simulink model "rectifiers"  (R2016a)
settings: Solver=ode4  StartTime=0.0  StopTime=2  FixedStep=1e-5  RelTol=1e-3
undefined symbols (not defined in the file): D1, lagging, pulse
libraries: powerlib x34, powerlib_meascontrol x20
settings Model: Creator=ugurm  LastModifiedBy=mesutto
settings DataIOCC: LimitDataPoints=on  SaveFormat=Array
settings DebuggingCC: UnderspecifiedInitializationDetection=Classic  MergeDetectMultiDrivingBlocksExec=none  SolverPrmCheckMsg=warning  StateNameClashWarn=warning
settings HardwareCC: ProdBitPerPointer=32  ProdLargestAtomicFloat=None  ProdIntDivRoundTo=Undefined  ProdEndianess=Unspecified  ProdWordSize=32  ProdHWDeviceType=32-bit Generic
settings ModelReferenceCC: PropagateSignalLabelsOutOfModel=off
settings ConfigComp: CovModelRefEnable=Off

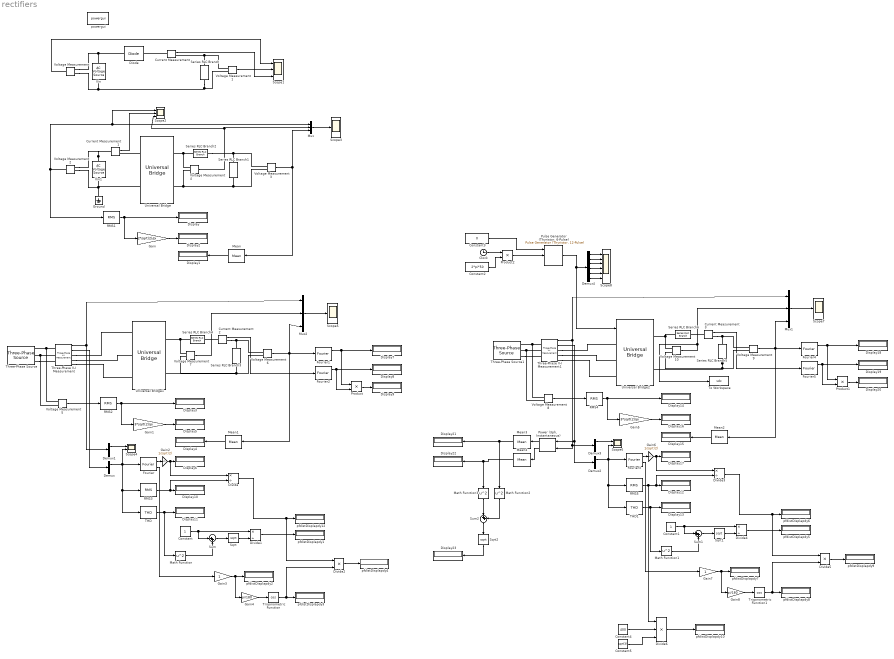
== system rectifiers ==
  Clock : Clock
  Constant : Constant
  Constant1 : Constant
  Constant2 : Constant  Value=2*pi*50
  Constant3 : Constant  Value=0
  Constant4 : Constant  Value=400
  Constant5 : Constant  Value=sqrt(3)
  Current Measurement{,1..3} (4 alike) : powerlib/Measurements/Current Measurement  PhasorSimulation=off  OutputType=Complex  PSBequivalent=0
  Demux{,1..3} (4 alike) : Demux  Outputs=3
  Demux4 : Demux  Outputs=6
  Diode : powerlib/Power Electronics/Diode  Ron=0.001  Lon=0  Vf=0.8  IC=0  UseSnubber=off  Rs=1e9  Cs=250e-9  Measurements=off
  Display{,1..23} (24 alike) : Display
  Divide{,1,3..4} (4 alike) : Product  Inputs=*/
  Divide2 : Product  Inputs=**
  Divide5 : Product  Inputs=**
  Divide6 : Product  Inputs=***
  Fourier : powerlib_meascontrol/Measurements/Fourier  Freq=50  n=1  InInit=[0, 0]  Ts=0
  Fourier{1..2,4..5} (4 alike) : powerlib_meascontrol/Measurements/Fourier  Freq=50  n=0  InInit=[0, 0]  Ts=0
  Fourier3 : powerlib_meascontrol/Measurements/Fourier  Freq=50  n=1  InInit=[0, 0]  Ts=0
  Gain : Gain  Gain=2*sqrt(2)/pi
  Gain1 : Gain  Gain=3*sqrt(2)/pi
  Gain2 : Gain  Gain=1/sqrt(2)
  Gain3 : Gain
  Gain4 : Gain  Gain=pi/180
  Gain5 : Gain  Gain=3*sqrt(2)/pi
  Gain6 : Gain  Gain=1/sqrt(2)
  Gain7 : Gain
  Gain8 : Gain  Gain=pi/180
  Ground : powerlib/Elements/Ground  LConnTagsString=a
  Math Function{,1..3} (4 alike) : Math  Operator=square  SaturateOnIntegerOverflow=on
  Mean{,1..4} (5 alike) : powerlib_meascontrol/Measurements/Mean  Freq=50  Vinit=0  Ts=0
  Mux : Mux  Inputs=3
  Mux1 : Mux  Inputs=3
  Mux2 : Mux  Inputs=3
  "Power (3ph, Instantaneous)" : powerlib_meascontrol/Measurements/Power (3ph, Instantaneous)
  Product : Product
  Product1 : Product
  Product2 : Product
  "Pulse Generator (Thyristor, 6-Pulse)" : powerlib_meascontrol/Pulse & Signal Generators/Pulse Generator (Thyristor, 12-Pulse)  GenType=6-pulse  Delta=D1 (lagging)  pwidth=60  Double_Pulse=off  Ts=0
  RMS{1..5} (5 alike) : powerlib_meascontrol/Measurements/RMS  TrueRMS=on  Freq=50  RMSInit=0  Ts=0
  Scope1 : Scope  NumInputPorts=3
  Scope2 : Scope  NumInputPorts=3
  Scope3 : Scope
  Scope4 : Scope  NumInputPorts=2
  Scope5 : Scope
  Scope6 : Scope  NumInputPorts=2
  Scope7 : Scope
  Scope8 : Scope  NumInputPorts=6
  Series RLC Branch : powerlib/Elements/Series RLC Branch  LConnTagsString=__new0  RConnTagsString=__new0  BranchType=RL  Resistance=2  Inductance=1/(2*pi*50)  SetiL0=off  InitialCurrent=0  Capacitance=1e-6  Setx0=off  InitialVoltage=0  Measurements=None
  Series RLC Branch1 : powerlib/Elements/Series RLC Branch  LConnTagsString=__new0  RConnTagsString=__new0  BranchType=R  Resistance=2  Inductance=1/(2*pi*50)  SetiL0=off  InitialCurrent=0  Capacitance=1e-6  Setx0=off  InitialVoltage=0  Measurements=None
  Series RLC Branch2 : powerlib/Elements/Series RLC Branch  LConnTagsString=__new0  RConnTagsString=__new0  BranchType=L  Resistance=2  Inductance=100/(2*pi*50)  SetiL0=off  InitialCurrent=0  Capacitance=1e-6  Setx0=off  InitialVoltage=0  Measurements=None
  Series RLC Branch3 : powerlib/Elements/Series RLC Branch  LConnTagsString=__new0  RConnTagsString=__new0  BranchType=R  Resistance=54  Inductance=1/(2*pi*50)  SetiL0=off  InitialCurrent=0  Capacitance=1e-6  Setx0=off  InitialVoltage=0  Measurements=None
  Series RLC Branch4 : powerlib/Elements/Series RLC Branch  LConnTagsString=__new0  RConnTagsString=__new0  BranchType=L  Resistance=2  Inductance=100/(2*pi*50)  SetiL0=off  InitialCurrent=0  Capacitance=1e-6  Setx0=off  InitialVoltage=0  Measurements=None
  Series RLC Branch5 : powerlib/Elements/Series RLC Branch  LConnTagsString=__new0  RConnTagsString=__new0  BranchType=R  Resistance=5  Inductance=1/(2*pi*50)  SetiL0=off  InitialCurrent=0  Capacitance=1e-6  Setx0=off  InitialVoltage=0  Measurements=None
  Series RLC Branch6 : powerlib/Elements/Series RLC Branch  LConnTagsString=__new0  RConnTagsString=__new0  BranchType=L  Resistance=2  Inductance=100/(2*pi*50)  SetiL0=off  InitialCurrent=0  Capacitance=1e-6  Setx0=off  InitialVoltage=0  Measurements=None
  Sqrt : Sqrt  SaturateOnIntegerOverflow=on
  Sqrt1 : Sqrt  SaturateOnIntegerOverflow=on
  Sqrt2 : Sqrt  SaturateOnIntegerOverflow=on
  Sum : Sum  Inputs=|++
  Sum1 : Sum  Inputs=|++
  Sum2 : Sum  Inputs=|++
  THD : powerlib_meascontrol/Measurements/THD  Freq=50  Ts=0
  THD1 : powerlib_meascontrol/Measurements/THD  Freq=50  Ts=0
  Three-Phase V-I Measurement : powerlib/Measurements/Three-Phase V-I Measurement  VoltageMeasurement=phase-to-ground  SetLabelV=off  LabelV=Vabc  Vpu=off  VpuLL=off  CurrentMeasurement=yes  SetLabelI=off  LabelI=Iabc  Ipu=off  Pbase=100e6  Vbase=500e3  OutputType=Complex  PhasorSimulation=off  PSBequivalent=0
  Three-Phase V-I Measurement1 : powerlib/Measurements/Three-Phase V-I Measurement  VoltageMeasurement=phase-to-ground  SetLabelV=off  LabelV=Vabc  Vpu=off  VpuLL=off  CurrentMeasurement=yes  SetLabelI=off  LabelI=Iabc  Ipu=off  Pbase=100e6  Vbase=500e3  OutputType=Complex  PhasorSimulation=off  PSBequivalent=0
  Three-Phase Source : powerlib/Electrical Sources/Three-Phase Source  InternalConnection=Yg  VoltagePhases=off  Voltage=400  PhaseAngle=0  Voltage_phases=[25e3 25e3 25e3]/sqrt(3)  PhaseAngles_phases=[0 -120 +120]  Frequency=50  NonIdealSource=off  SpecifyImpedance=off  Resistance=0.8929  Inductance=16.58e-3  ShortCircuitLevel=100e6  BaseVoltage=25e3  XRratio=7  BusType=swing  Pref=10e3  Qref=0  Prefabc=[10e3, 10e3, 10e3]  Qrefabc=[0, 0, 0]  Qmin=-inf  Qmax=inf
  Three-Phase Source1 : powerlib/Electrical Sources/Three-Phase Source  InternalConnection=Yg  VoltagePhases=off  Voltage=400  PhaseAngle=0  Voltage_phases=[25e3 25e3 25e3]/sqrt(3)  PhaseAngles_phases=[0 -120 +120]  Frequency=50  NonIdealSource=off  SpecifyImpedance=off  Resistance=0.8929  Inductance=16.58e-3  ShortCircuitLevel=100e6  BaseVoltage=25e3  XRratio=7  BusType=swing  Pref=10e3  Qref=0  Prefabc=[10e3, 10e3, 10e3]  Qrefabc=[0, 0, 0]  Qmin=-inf  Qmax=inf
  To Workspace : ToWorkspace  VariableName=vdc  SaveFormat=Structure With Time  SampleTime=-1
  Trigonometric Function : Trigonometry  Operator=cos
  Trigonometric Function1 : Trigonometry  Operator=cos
  Universal Bridge : powerlib/Power Electronics/Universal Bridge  Arms=2  SnubberResistance=1e5  SnubberCapacitance=inf  Device=Diodes  Ron=1e-3  Lon=0  ForwardVoltages="[  0  0  ]"  ForwardVoltage=0  GTOparameters=[ 10e-6 , 20e-6 ]  IGBTparameters=[ 1e-6 , 2e-6 ]  Measurements=None  Measurements_2=None  converterType=Rectifier
  Universal Bridge1 : powerlib/Power Electronics/Universal Bridge  Arms=3  SnubberResistance=1e5  SnubberCapacitance=inf  Device=Diodes  Ron=1e-3  Lon=0  ForwardVoltages="[  0  0  ]"  ForwardVoltage=0  GTOparameters=[ 10e-6 , 20e-6 ]  IGBTparameters=[ 1e-6 , 2e-6 ]  Measurements=None  Measurements_2=None  converterType=Rectifier
  Universal Bridge2 : powerlib/Power Electronics/Universal Bridge  Arms=3  SnubberResistance=1e5  SnubberCapacitance=inf  Device=Thyristors  Ron=1e-3  Lon=0  ForwardVoltages="[  0  0  ]"  ForwardVoltage=0  GTOparameters=[ 10e-6 , 20e-6 ]  IGBTparameters=[ 1e-6 , 2e-6 ]  Measurements=None  Measurements_2=None  converterType=Rectifier
  Vin : powerlib/Electrical Sources/AC Voltage Source  Amplitude=230*sqrt(2)  Phase=0  Frequency=50  SampleTime=0  Measurements=None  BusType=swing  Pref=10e3  Qref=0  Qmin=-inf  Qmax=+inf
  Vin1 : powerlib/Electrical Sources/AC Voltage Source  Amplitude=230*sqrt(2)  Phase=0  Frequency=50  SampleTime=0  Measurements=None  BusType=swing  Pref=10e3  Qref=0  Qmin=-inf  Qmax=+inf
  Voltage Measurement{,1..10} (11 alike) : powerlib/Measurements/Voltage Measurement  PhasorSimulation=off  OutputType=Complex  PSBequivalent=0
  pfdistDisplapdy{1..10,12} (11 alike) : Display
  powergui : powerlib/powergui  Priority=1  SimulationMode=Discrete  SolverType=Tustin/Backward Euler (TBE)  SampleTime=1e-5  frequency=60  SPID=off  DisableSnubberDevices=off  DisableRonSwitches=off  DisableVfSwitches=off  SwTol=0  DisplayEquations=off  Interpol=off  ExternalGateDelay=off  methode=off  Ts=10  FunctionMessages=off  echomessages=off  HookPort=off  EnableUseOfTLC=off  x0status=blocks  frequencyindice=50  Pbase=100e6  ErrMax=1e-4  Iterations=50  UnitsV=kV  UnitsW=MW  buscounter=0  RestoreLinks=warning  ResistiveCurrentMeasurement=off  Frange=[0:2:500]  Ylog=off  Xlog=on  ShowGrid=off  save=off  variable=ZData  structure=vdc  ZoomFFT=off  StartTime=0.2  cycles=20  DisplayStyle=5  fundamental=50  FreqAxis=off  MaxFrequency=2000  frequencyindicesteady=1  RmsSteady=1  display=off
  wires:
  Voltage Measurement/1 -> Scope1/1
  Voltage Measurement1/1 -> Scope1/2
  Current Measurement/1 -> Scope1/3
  Voltage Measurement2/1 -> Scope2/1, Mux/1, RMS1/1
  Voltage Measurement4/1 -> Scope2/3, Mux/2
  Voltage Measurement3/1 -> Mux/3, Mean/1
  Mux/1 -> Scope3/1
  RMS1/1 -> Gain/1, Display/1
  Current Measurement1/1 -> Scope2/2
  Mean/1 -> Display1/1
  Gain/1 -> Display2/1
  Voltage Measurement6/1 -> Mux2/3, Mean1/1, Fourier1/1
  RMS2/1 -> Gain1/1, Display3/1
  Mean1/1 -> Display4/1
  Gain1/1 -> Display5/1
  Three-Phase V-I Measurement/1 -> Demux1/1, Mux2/1
  Voltage Measurement7/1 -> Mux2/2
  Mux2/1 -> Scope5/1
  Voltage Measurement5/1 -> RMS2/1
  Three-Phase V-I Measurement/2 -> Demux/1
  Demux/1 -> THD/1, RMS3/1, Scope4/2, Fourier/1
  Fourier/1 -> Gain2/1
  Current Measurement2/1 -> Fourier2/1
  Fourier1/1 -> Product/1, Display7/1
  Fourier2/1 -> Product/2, Display8/1
  Product/1 -> Display9/1
  Demux1/1 -> Scope4/1
  RMS3/1 -> Divide/2, Display10/1
  Gain2/1 -> Divide/1, Display6/1
  THD/1 -> Math Function/1, Display11/1
  Divide/1 -> Divide2/1, pfdistDisplapdy12/1
  Constant/1 -> Sum/1, Divide1/1
  Sqrt/1 -> Divide1/2
  Math Function/1 -> Sum/2
  Sum/1 -> Sqrt/1
  Divide1/1 -> pfdistDisplapdy1/1
  Fourier/2 -> Gain3/1
  Gain3/1 -> Gain4/1, pfdistDisplapdy2/1
  Trigonometric Function/1 -> Divide2/2, pfdistDisplapdy3/1
  Divide2/1 -> pfdistDisplapdy4/1
  Gain4/1 -> Trigonometric Function/1
  Voltage Measurement9/1 -> Mux1/3, Mean2/1, Fourier4/1
  RMS4/1 -> Gain5/1, Display14/1
  Mean2/1 -> Display15/1
  Gain5/1 -> Display16/1
  Three-Phase V-I Measurement1/1 -> "Power (3ph, Instantaneous)"/1, Demux3/1, Mux1/1
  Voltage Measurement10/1 -> To Workspace/1, Mux1/2
  Mux1/1 -> Scope7/1
  Voltage Measurement8/1 -> RMS4/1
  Three-Phase V-I Measurement1/2 -> Demux2/1, "Power (3ph, Instantaneous)"/2
  Demux2/1 -> THD1/1, RMS5/1, Scope6/2, Fourier3/1
  Fourier3/1 -> Gain6/1
  Current Measurement3/1 -> Fourier5/1
  Fourier4/1 -> Product1/1, Display18/1
  Fourier5/1 -> Product1/2, Display19/1
  Product1/1 -> Display20/1
  Demux3/1 -> Scope6/1
  RMS5/1 -> Divide6/1, Divide3/2, Display12/1
  Gain6/1 -> Divide3/1, Display17/1
  THD1/1 -> Math Function1/1, Display13/1
  Divide3/1 -> Divide5/1, pfdistDisplapdy6/1
  Constant1/1 -> Sum1/1, Divide4/1
  Sqrt1/1 -> Divide4/2
  Math Function1/1 -> Sum1/2
  Sum1/1 -> Sqrt1/1
  Divide4/1 -> pfdistDisplapdy5/1
  Fourier3/2 -> Gain7/1
  Gain7/1 -> Gain8/1, pfdistDisplapdy7/1
  Trigonometric Function1/1 -> Divide5/2, pfdistDisplapdy8/1
  Divide5/1 -> pfdistDisplapdy9/1
  Gain8/1 -> Trigonometric Function1/1
  "Pulse Generator (Thyristor, 6-Pulse)"/1 -> Demux4/1, Universal Bridge2/1
  Product2/1 -> "Pulse Generator (Thyristor, 6-Pulse)"/2
  Clock/1 -> Product2/1
  Constant2/1 -> Product2/2
  Constant3/1 -> "Pulse Generator (Thyristor, 6-Pulse)"/1
  "Power (3ph, Instantaneous)"/2 -> Mean3/1
  "Power (3ph, Instantaneous)"/1 -> Mean4/1
  Mean3/1 -> Math Function2/1, Display21/1
  Mean4/1 -> Math Function3/1, Display22/1
  Constant5/1 -> Divide6/3
  Constant4/1 -> Divide6/2
  Math Function2/1 -> Sum2/2
  Math Function3/1 -> Sum2/1
  Sum2/1 -> Sqrt2/1
  Sqrt2/1 -> Display23/1
  Divide6/1 -> pfdistDisplapdy10/1
  Demux4/1 -> Scope8/1
  Demux4/3 -> Scope8/3
  Demux4/2 -> Scope8/2
  Demux4/4 -> Scope8/4
  Demux4/5 -> Scope8/5
  Demux4/6 -> Scope8/6
  connections:
  Diode/LConn1 -- Voltage Measurement/LConn1 -- Vin/RConn1
  Current Measurement/LConn1 -- Diode/RConn1
  Series RLC Branch/LConn1 -- Voltage Measurement1/LConn1 -- Current Measurement/RConn1
  Series RLC Branch/RConn1 -- Voltage Measurement1/LConn2 -- Voltage Measurement/LConn2 -- Vin/LConn1
  Vin1/RConn1 -- Current Measurement1/LConn1 -- Voltage Measurement2/LConn1
  Voltage Measurement3/LConn1 -- Series RLC Branch2/LConn1 -- Series RLC Branch1/LConn1
  Voltage Measurement4/LConn2 -- Universal Bridge/RConn2 -- Series RLC Branch1/RConn1 -- Voltage Measurement3/LConn2
  Voltage Measurement2/LConn2 -- Universal Bridge/LConn2 -- Vin1/LConn1 -- Ground/LConn1
  Universal Bridge/LConn1 -- Current Measurement1/RConn1
  Series RLC Branch2/RConn1 -- Universal Bridge/RConn1 -- Voltage Measurement4/LConn1
  Voltage Measurement6/LConn1 -- Current Measurement2/RConn1 -- Series RLC Branch3/LConn1
  Voltage Measurement6/LConn2 -- Voltage Measurement7/LConn2 -- Universal Bridge1/RConn2 -- Series RLC Branch3/RConn1
  Series RLC Branch4/RConn1 -- Universal Bridge1/RConn1 -- Voltage Measurement7/LConn1
  Three-Phase V-I Measurement/LConn1 -- Voltage Measurement5/LConn1 -- Three-Phase Source/RConn1
  Three-Phase Source/RConn2 -- Voltage Measurement5/LConn2 -- Three-Phase V-I Measurement/LConn2
  Three-Phase Source/RConn3 -- Three-Phase V-I Measurement/LConn3
  Three-Phase V-I Measurement/RConn1 -- Universal Bridge1/LConn1
  Three-Phase V-I Measurement/RConn2 -- Universal Bridge1/LConn2
  Three-Phase V-I Measurement/RConn3 -- Universal Bridge1/LConn3
  Current Measurement2/LConn1 -- Series RLC Branch4/LConn1
  Voltage Measurement9/LConn1 -- Current Measurement3/RConn1 -- Series RLC Branch5/LConn1
  Series RLC Branch5/RConn1 -- Voltage Measurement10/LConn2 -- Universal Bridge2/RConn2 -- Voltage Measurement9/LConn2
  Series RLC Branch6/RConn1 -- Voltage Measurement10/LConn1 -- Universal Bridge2/RConn1
  Three-Phase V-I Measurement1/LConn1 -- Voltage Measurement8/LConn1 -- Three-Phase Source1/RConn1
  Three-Phase Source1/RConn2 -- Voltage Measurement8/LConn2 -- Three-Phase V-I Measurement1/LConn2
  Three-Phase V-I Measurement1/RConn2 -- Universal Bridge2/LConn2
  Three-Phase V-I Measurement1/RConn1 -- Universal Bridge2/LConn1
  Current Measurement3/LConn1 -- Series RLC Branch6/LConn1
  Three-Phase Source1/RConn3 -- Three-Phase V-I Measurement1/LConn3
  Three-Phase V-I Measurement1/RConn3 -- Universal Bridge2/LConn3
